simulink model "mekf_static_test"  (R2018b)
settings: Solver=VariableStepAuto  StartTime=0.0  StopTime=5400.0  RelTol=1e-3
undefined symbols (not defined in the file or in its folder): fswParams, simParams
libraries: vrlib x2, aerolibutil x2, quat_err_lib x2, MEKF_lib x1, PD_Controller_Lib x1, gyroscope_lib x1, ss_angles_2_vec x1, sun_sensor_lib x1, two_norm x1, ss_vec_2_angles x1, quat_kinematics_lib x1, rigid_body_dynamics_lib x1
settings Model: Creator=Taylor  LastModifiedBy=Taylor

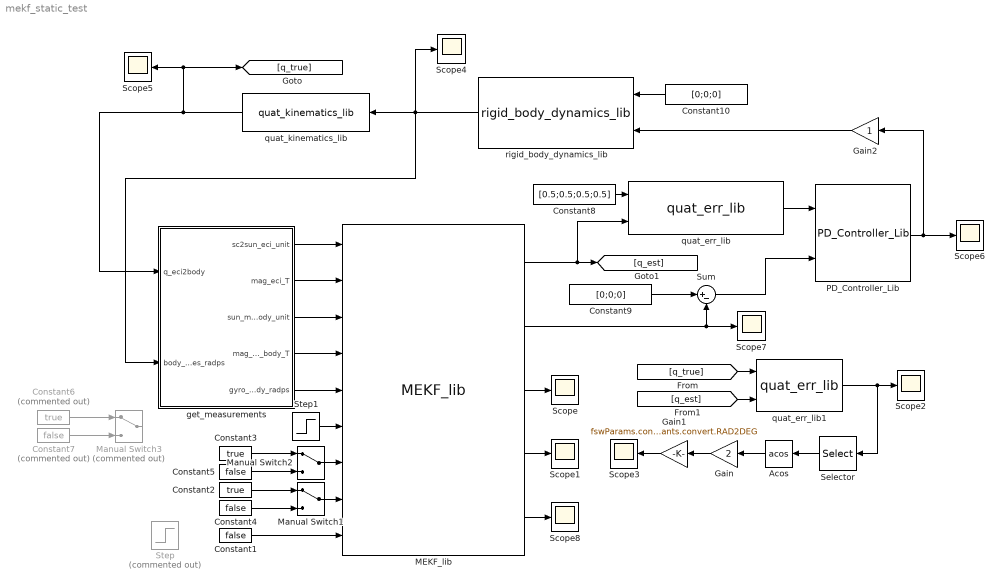
== system mekf_static_test ==
  Acos : Trigonometry  Operator=acos
  Constant1 : Constant  Value=false
  Constant10 : Constant  Value=[0;0;0]
  Constant2 : Constant  Value=true
  Constant3 : Constant  Value=true
  Constant4 : Constant  Value=false
  Constant5 : Constant  Value=false
  Constant6 : Constant  Commented=on  Value=true
  Constant7 : Constant  Commented=on  Value=false
  Constant8 : Constant  Value=[0.5;0.5;0.5;0.5]
  Constant9 : Constant  Value=[0;0;0]
  Gain : Gain  Gain=2
  Gain1 : Gain  Gain=fswParams.constants.convert.RAD2DEG
  Gain2 : Gain
  MEKF_lib : MEKF_lib/MEKF_lib  SystemSampleTime=-1
  Manual Switch1 : ManualSwitch
  Manual Switch2 : ManualSwitch
  Manual Switch3 : ManualSwitch  Commented=on
  PD_Controller_Lib : PD_Controller_Lib/PD_Controller_Lib  SystemSampleTime=-1
  Scope{,1..8} (9 alike) : Scope
  Selector : Selector  InputPortWidth=4  IndexOptions=Index vector (dialog)  Indices=[1]  OutputSizes=1
  Step : Step  Commented=on  Time=10  Before=1  After=0  SampleTime=0
  Step1 : Step  Time=30  SampleTime=0
  Sum : Sum  Inputs=|+-
  get_measurements : Subsystem
  quat_err_lib : quat_err_lib/quat_err_lib  SystemSampleTime=-1
  quat_err_lib1 : quat_err_lib/quat_err_lib  SystemSampleTime=-1
  quat_kinematics_lib : quat_kinematics_lib/quat_kinematics_lib  SystemSampleTime=-1
  rigid_body_dynamics_lib : rigid_body_dynamics_lib/rigid_body_dynamics_lib  SystemSampleTime=-1
  wires:
  Constant4/1 -> Manual Switch1/2
  Constant2/1 -> Manual Switch1/1
  Manual Switch1/1 -> MEKF_lib/8
  Constant3/1 -> Manual Switch2/1
  Constant5/1 -> Manual Switch2/2
  Constant7/1 -> Manual Switch3/2
  Constant6/1 -> Manual Switch3/1
  Manual Switch2/1 -> MEKF_lib/7
  rigid_body_dynamics_lib/1 -> Scope4/1, get_measurements/2(body_rates_radps), quat_kinematics_lib/1
  MEKF_lib/1 -> [q_est], quat_err_lib/2
  quat_err_lib/1 -> PD_Controller_Lib/1
  Constant8/1 -> quat_err_lib/1
  Constant9/1 -> Sum/1
  MEKF_lib/2 -> Scope7/1, Sum/2
  Sum/1 -> PD_Controller_Lib/2
  PD_Controller_Lib/1 -> Scope6/1, Gain2/1
  Constant10/1 -> rigid_body_dynamics_lib/1
  get_measurements/1("sc2sun_eci_unit ") -> MEKF_lib/1
  get_measurements/5(gyro_meas_body_radps) -> MEKF_lib/5
  get_measurements/4(mag_meas_body_T) -> MEKF_lib/4
  get_measurements/3(sun_meas_body_unit) -> MEKF_lib/3
  get_measurements/2(mag_eci_T) -> MEKF_lib/2
  quat_kinematics_lib/1 -> [q_true], Scope5/1, get_measurements/1(q_eci2body)
  MEKF_lib/3 -> Scope/1
  MEKF_lib/4 -> Scope1/1
  [q_true] -> quat_err_lib1/1
  [q_est] -> quat_err_lib1/2
  quat_err_lib1/1 -> Selector/1, Scope2/1
  Selector/1 -> Acos/1
  Gain/1 -> Gain1/1
  Gain1/1 -> Scope3/1
  Acos/1 -> Gain/1
  MEKF_lib/5 -> Scope8/1
  Gain2/1 -> rigid_body_dynamics_lib/2
  Step1/1 -> MEKF_lib/6
  Constant1/1 -> MEKF_lib/9

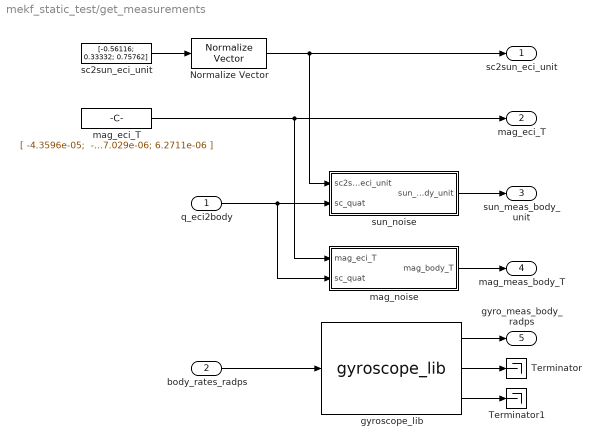
== system mekf_static_test/get_measurements ==
  q_eci2body : Inport
  body_rates_radps : Inport  Port=2
  Normalize Vector : vrlib/Utilities/Normalize Vector  maxzero=0
      settings: SourceProductName=Simulink 3D Animation  SourceProductBaseCode=VR
  Terminator : Terminator
  Terminator1 : Terminator
  gyroscope_lib : gyroscope_lib/gyroscope_lib  id_s=1
  "mag_eci_T " : Constant  Value="[ -4.3596e-05;  -7.029e-06; 6.2711e-06 ]"
  mag_noise : Subsystem
  sc2sun_eci_unit : Constant  Value=|
      | [-0.56116;
      |       0.33332;
      |       0.75762]
  sun_noise : Subsystem
  "sc2sun_eci_unit " : Outport
  mag_eci_T : Outport  Port=2
  sun_meas_body_unit : Outport  Port=3
  mag_meas_body_T : Outport  Port=4
  gyro_meas_body_radps : Outport  Port=5
  wires:
  sc2sun_eci_unit/1 -> Normalize Vector/1
  q_eci2body/1 -> mag_noise/2(sc_quat), sun_noise/2(sc_quat)
  gyroscope_lib/2 -> Terminator/1
  gyroscope_lib/3 -> Terminator1/1
  body_rates_radps/1 -> gyroscope_lib/1
  gyroscope_lib/1 -> gyro_meas_body_radps/1
  sun_noise/1(sun_meas_body_unit) -> sun_meas_body_unit/1
  mag_noise/1(mag_body_T) -> mag_meas_body_T/1
  "mag_eci_T "/1 -> mag_noise/1(mag_eci_T), mag_eci_T/1
  Normalize Vector/1 -> sun_noise/1(sc2sun_eci_unit), "sc2sun_eci_unit "/1

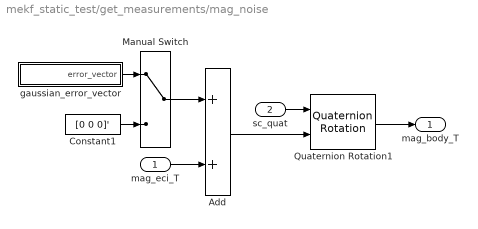
== system mekf_static_test/get_measurements/mag_noise ==
  mag_eci_T : Inport
  sc_quat : Inport  Port=2
  Add : Sum
  Constant1 : Constant  Value=[0 0 0]'
  Manual Switch : ManualSwitch
  Quaternion Rotation1 : aerolibutil/Quaternion Rotation
  gaussian_error_vector : Subsystem
  mag_body_T : Outport
  wires:
  sc_quat/1 -> Quaternion Rotation1/1
  Quaternion Rotation1/1 -> mag_body_T/1
  gaussian_error_vector/1(error_vector) -> Manual Switch/1
  Constant1/1 -> Manual Switch/2
  mag_eci_T/1 -> Add/2
  Manual Switch/1 -> Add/1
  Add/1 -> Quaternion Rotation1/2

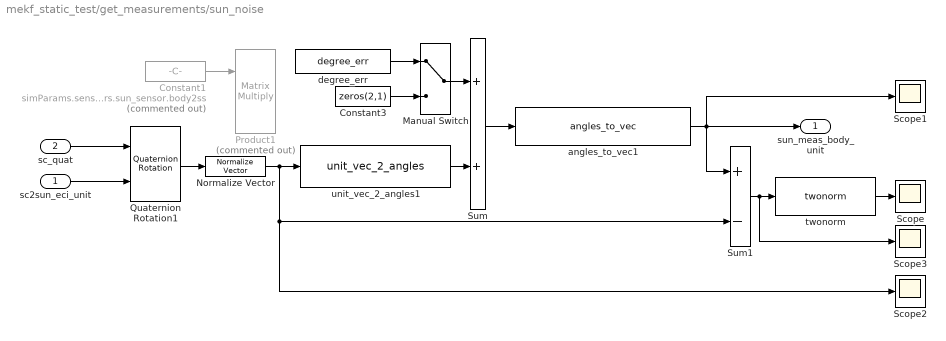
== system mekf_static_test/get_measurements/sun_noise ==
  sc2sun_eci_unit : Inport
  sc_quat : Inport  Port=2
  Constant1 : Constant  Commented=on  Value=simParams.sensors.sun_sensor.body2ss
  Constant3 : Constant  Value=zeros(2,1)
  Manual Switch : ManualSwitch
  Normalize Vector : vrlib/Utilities/Normalize Vector  maxzero=0
      settings: SourceProductName=Simulink 3D Animation  SourceProductBaseCode=VR
  Product1 : Product  Commented=on  Multiplication=Matrix(*)  RndMeth=Zero
  Quaternion Rotation1 : aerolibutil/Quaternion Rotation
  Scope{,1..3} (4 alike) : Scope
  Sum : Sum
  Sum1 : Sum  Inputs=+-
  angles_to_vec1 : ss_angles_2_vec/angles_to_vec  SystemSampleTime=-1
  degree_err : sun_sensor_lib/sun_sensor_lib /degree_err  SystemSampleTime=-1
  twonorm : two_norm/twonorm  SystemSampleTime=-1
  unit_vec_2_angles1 : ss_vec_2_angles/unit_vec_2_angles  SystemSampleTime=-1
  sun_meas_body_unit : Outport
  wires:
  angles_to_vec1/1 -> Scope1/1, sun_meas_body_unit/1, Sum1/1
  sc2sun_eci_unit/1 -> Quaternion Rotation1/2
  sc_quat/1 -> Quaternion Rotation1/1
  Quaternion Rotation1/1 -> Normalize Vector/1
  Normalize Vector/1 -> unit_vec_2_angles1/1, Sum1/2, Scope2/1
  degree_err/1 -> Manual Switch/1
  Constant3/1 -> Manual Switch/2
  Manual Switch/1 -> Sum/1
  Constant1/1 -> Product1/1
  unit_vec_2_angles1/1 -> Sum/2
  twonorm/1 -> Scope/1
  Sum1/1 -> twonorm/1, Scope3/1
  Sum/1 -> angles_to_vec1/1

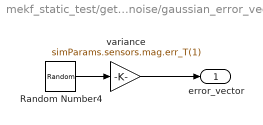
== system mekf_static_test/get_measurements/mag_noise/gaussian_error_vector ==
  Random Number4 : RandomNumber  Mean=[0;0;0]  Variance=[1;1;1]  Seed=[1;2;3]  SampleTime=simParams.sensors.mag.sample_time_s
  variance : Gain  Gain=simParams.sensors.mag.err_T(1)
  error_vector : Outport
  wires:
  variance/1 -> error_vector/1
  Random Number4/1 -> variance/1
